simulink model "Copy_of_chap12_2sim"  (Simulink 10.3)
settings: Solver=FixedStepAuto  StartTime=0.0  StopTime=10  FixedStep=0.000001  RelTol=1e-3  EnableMultiTasking=on
settings Model: Creator=ljk  LastModifiedBy=fu  ExtModeTrigMode=oneshot  ExtModeArmWhenConnect=off
settings OptimizationCC: BlockReduction=off  BooleanDataType=off
settings DebuggingCC: SaveWithParameterizedLinksMsg=none  SignalResolutionControl=TryResolveAllWithWarning  MultiTaskDSMMsg=warning  MultiTaskCondExecSysMsg=none
settings HardwareCC: TargetUnknown=on

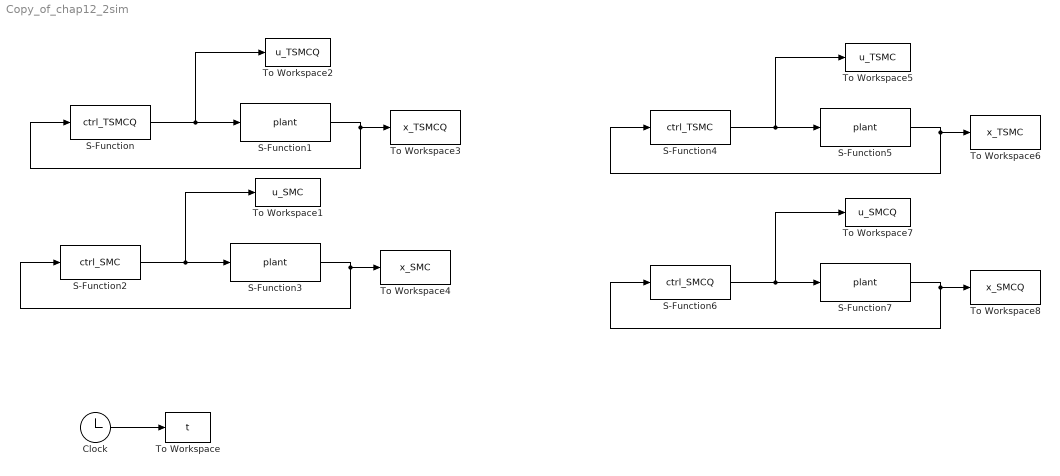
== system Copy_of_chap12_2sim ==
  Clock : Clock
  S-Function : S-Function  FunctionName=ctrl_TSMCQ  SFunctionDeploymentMode=off  EnableBusSupport=off
  S-Function{1,3,5,7} (4 alike) : S-Function  FunctionName=plant  SFunctionDeploymentMode=off  EnableBusSupport=off
  S-Function2 : S-Function  FunctionName=ctrl_SMC  SFunctionDeploymentMode=off  EnableBusSupport=off
  S-Function4 : S-Function  FunctionName=ctrl_TSMC  SFunctionDeploymentMode=off  EnableBusSupport=off
  S-Function6 : S-Function  FunctionName=ctrl_SMCQ  SFunctionDeploymentMode=off  EnableBusSupport=off
  To Workspace : ToWorkspace  VariableName=t  SampleTime=-1
  To Workspace1 : ToWorkspace  VariableName=u_SMC  SampleTime=-1
  To Workspace2 : ToWorkspace  VariableName=u_TSMCQ  SampleTime=-1
  To Workspace3 : ToWorkspace  VariableName=x_TSMCQ  SampleTime=-1
  To Workspace4 : ToWorkspace  VariableName=x_SMC  SampleTime=-1
  To Workspace5 : ToWorkspace  VariableName=u_TSMC  SampleTime=-1
  To Workspace6 : ToWorkspace  VariableName=x_TSMC  SampleTime=-1
  To Workspace7 : ToWorkspace  VariableName=u_SMCQ  SampleTime=-1
  To Workspace8 : ToWorkspace  VariableName=x_SMCQ  SampleTime=-1
  wires:
  S-Function/1 -> S-Function1/1, To Workspace2/1
  Clock/1 -> To Workspace/1
  S-Function1/1 -> To Workspace3/1, S-Function/1
  S-Function3/1 -> To Workspace4/1, S-Function2/1
  S-Function2/1 -> S-Function3/1, To Workspace1/1
  S-Function4/1 -> S-Function5/1, To Workspace5/1
  S-Function5/1 -> To Workspace6/1, S-Function4/1
  S-Function6/1 -> S-Function7/1, To Workspace7/1
  S-Function7/1 -> To Workspace8/1, S-Function6/1
